simulink model "lab5_2"  (R2018a)
settings: Solver=ode45  StartTime=0.0  StopTime=15  MaxStep=0.001  RelTol=1e-3
values from neighbouring files (symbols this model uses):
  A10 = Ak    [modele05.m]
  A100 = Ak    [modele05.m]
  A15000 = Ak    [modele05.m]
  A30 = Ak    [modele05.m]
  A5 = Ak    [modele05.m]
  B = [ 0 ; 0 ]    [modele05.m]
  C = [ 1 0 ; 0 1]    [modele05.m]
  D = [ 0 ; 0]    [modele05.m]
settings Model: Creator=Koala  LastModifiedBy=Koala

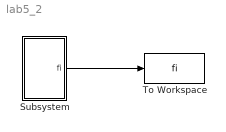
== system lab5_2 ==
  Subsystem : Subsystem  mask{m=2, k=2, g=9.81, l=1, fi0=90}
  To Workspace : ToWorkspace  VariableName=fi  SampleTime=-1
  wires:
  Subsystem/1(fi) -> To Workspace/1

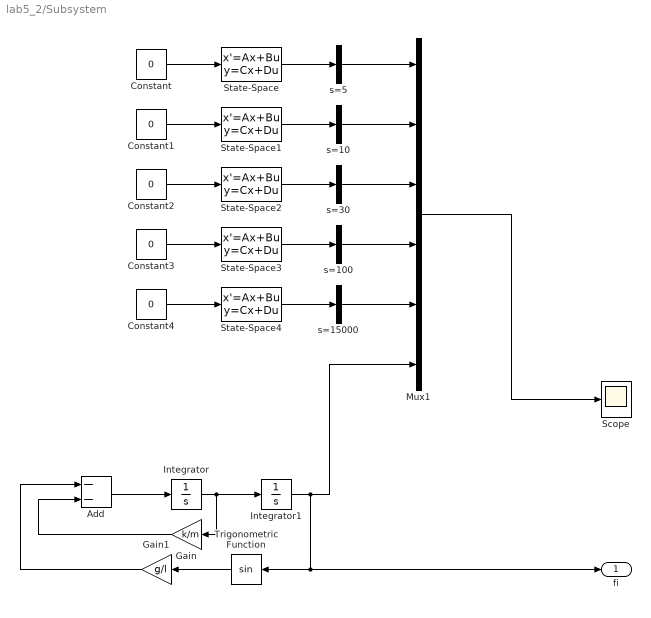
== system lab5_2/Subsystem ==
  Add : Sum  Inputs=--
  Constant{,1..4} (5 alike) : Constant  Value=0
  Gain : Gain  Gain=k/m
  Gain1 : Gain  Gain=g/l
  Integrator : Integrator
  Integrator1 : Integrator  InitialCondition=fi0*pi/180
  Mux1 : Mux  Inputs=6
  Scope : Scope
  State-Space : StateSpace  A=A5  B=B  C=C  D=D  InitialCondition=[pi/2 0]
  State-Space1 : StateSpace  A=A10  B=B  C=C  D=D  InitialCondition=[pi/2 0]
  State-Space2 : StateSpace  A=A30  B=B  C=C  D=D  InitialCondition=[pi/2 0]
  State-Space3 : StateSpace  A=A100  B=B  C=C  D=D  InitialCondition=[pi/2 0]
  State-Space4 : StateSpace  A=A15000  B=B  C=C  D=D  InitialCondition=[pi/2 0]
  Trigonometric Function : Trigonometry
  "s=10 " : Demux  Outputs=1
  s=100 : Demux  Outputs=1
  s=15000 : Demux  Outputs=1
  "s=30 " : Demux  Outputs=1
  "s=5 " : Demux  Outputs=1
  fi : Outport
  wires:
  Gain/1 -> Add/2
  Add/1 -> Integrator/1
  Integrator/1 -> Gain/1, Integrator1/1
  Trigonometric Function/1 -> Gain1/1
  Gain1/1 -> Add/1
  Mux1/1 -> Scope/1
  Integrator1/1 -> Mux1/6, fi/1, Trigonometric Function/1
  "s=30 "/1 -> Mux1/3
  s=15000/1 -> Mux1/5
  s=100/1 -> Mux1/4
  "s=5 "/1 -> Mux1/1
  "s=10 "/1 -> Mux1/2
  Constant3/1 -> State-Space3/1
  Constant2/1 -> State-Space2/1
  State-Space2/1 -> "s=30 "/1
  Constant/1 -> State-Space/1
  Constant4/1 -> State-Space4/1
  Constant1/1 -> State-Space1/1
  State-Space/1 -> "s=5 "/1
  State-Space1/1 -> "s=10 "/1
  State-Space3/1 -> s=100/1
  State-Space4/1 -> s=15000/1
